simulink model "versionAnaliticaPunto2a"  (R2017b)
settings: Solver=VariableStepAuto  StartTime=0.0  StopTime=0.001  RelTol=1e-3
settings Model: Creator=user  LastModifiedBy=user

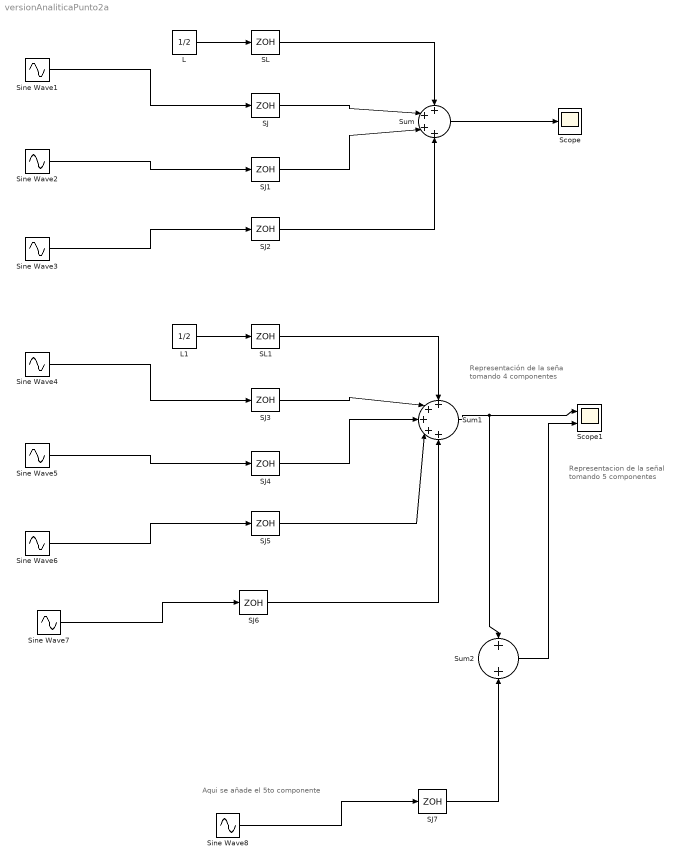
== system versionAnaliticaPunto2a ==
  note: Representacion de la señal
      |  tomando 5 componentes
  note: Representación de la seña tomando 4 componentes
  note: Aqui se añade el 5to componente
  L : Constant  Value=1/2  SampleTime=1/(6*(1000*2*pi))
  L1 : Constant  Value=1/2  SampleTime=1/(6*(1000*2*pi))
  SJ{,1..7} (8 alike) : ZeroOrderHold  SampleTime=1/(10*100e3)
  SL : ZeroOrderHold  SampleTime=1/(10*100e3)
  SL1 : ZeroOrderHold  SampleTime=1/(10*100e3)
  Scope : Scope
  Scope1 : Scope  NumInputPorts=2
  Sine Wave1 : Sin  Amplitude=0.6366  Frequency=10e3*2*pi  SampleTime=0
      settings: AttributesFormatString=|
      | Frecuency = %<Frequency>
      | Phase = %<Phase>
  Sine Wave2 : Sin  Amplitude=0.2122  Frequency=3*10e3*2*pi  SampleTime=0
      settings: AttributesFormatString=|
      | Frecuency = %<Frequency>
      | Phase = %<Phase>
  Sine Wave3 : Sin  Amplitude=0.127  Frequency=5*10e3*2*pi  SampleTime=0
      settings: AttributesFormatString=|
      | Frecuency = %<Frequency>
      | Phase = %<Phase>
  Sine Wave4 : Sin  Amplitude=0.6366  Frequency=10e3*2*pi  SampleTime=0
      settings: AttributesFormatString=|
      | Frecuency = %<Frequency>
      | Phase = %<Phase>
  Sine Wave5 : Sin  Amplitude=0.2122  Frequency=3*10e3*2*pi  SampleTime=0
      settings: AttributesFormatString=|
      | Frecuency = %<Frequency>
      | Phase = %<Phase>
  Sine Wave6 : Sin  Amplitude=0.127  Frequency=5*10e3*2*pi  SampleTime=0
      settings: AttributesFormatString=|
      | Frecuency = %<Frequency>
      | Phase = %<Phase>
  Sine Wave7 : Sin  Amplitude=0.0909  Frequency=7*10e3*2*pi  SampleTime=0
      settings: AttributesFormatString=|
      | Frecuency = %<Frequency>
      | Phase = %<Phase>
  Sine Wave8 : Sin  Amplitude=0.0707  Frequency=9*10e3*2*pi  SampleTime=0
      settings: AttributesFormatString=|
      | Frecuency = %<Frequency>
      | Phase = %<Phase>
  Sum : Sum  Inputs=+|+|+|+
  Sum1 : Sum  Inputs=+|+|+|+|+
  Sum2 : Sum  Inputs=+|+
  wires:
  SL/1 -> Sum/1
  SJ/1 -> Sum/2
  SJ1/1 -> Sum/3
  SJ2/1 -> Sum/4
  L/1 -> SL/1
  Sine Wave1/1 -> SJ/1
  Sine Wave2/1 -> SJ1/1
  Sine Wave3/1 -> SJ2/1
  Sum/1 -> Scope/1
  SJ5/1 -> Sum1/4
  L1/1 -> SL1/1
  Sine Wave5/1 -> SJ4/1
  SL1/1 -> Sum1/1
  SJ4/1 -> Sum1/3
  Sine Wave4/1 -> SJ3/1
  Sine Wave6/1 -> SJ5/1
  SJ3/1 -> Sum1/2
  Sum1/1 -> Sum2/1, Scope1/1
  Sine Wave7/1 -> SJ6/1
  SJ6/1 -> Sum1/5
  Sine Wave8/1 -> SJ7/1
  SJ7/1 -> Sum2/2
  Sum2/1 -> Scope1/2
